simulink model "dual_hall_ideal_sincos"  (R2024b)
settings: Solver=ode4  StartTime=0.0  StopTime=hall_t_stop_s  FixedStep=hall_ts_sim_s  RelTol=1e-3
model workspace (MAT data in the model file):
  hall_adc_bits = 16
  hall_amp_c_v = 0.85
  hall_amp_s_v = 1
  hall_amp_v = 1
  hall_f_mag_hz = 3
  hall_f_mech_hz = 0.5
  hall_magnet_od_mm = 18
  hall_mech_speed_rpm = 30
  hall_offset_c_actual_v = 1.57
  hall_offset_err_c_v = -0.08
  hall_offset_err_s_v = 0.05
  hall_offset_s_actual_v = 1.7
  hall_offset_v = 1.65
  hall_omega_mech_rad_s = 3.14159265359
  hall_phase_err_deg = 5
  hall_phase_err_rad = 0.0872664625997
  hall_pole_pairs = 6
  hall_t_stop_s = 2
  hall_theta0_rad = 0
  hall_ts_sim_s = 0.0001
  hall_vref_v = 3.3
settings Model: Creator=26683  LastModifiedBy=26683

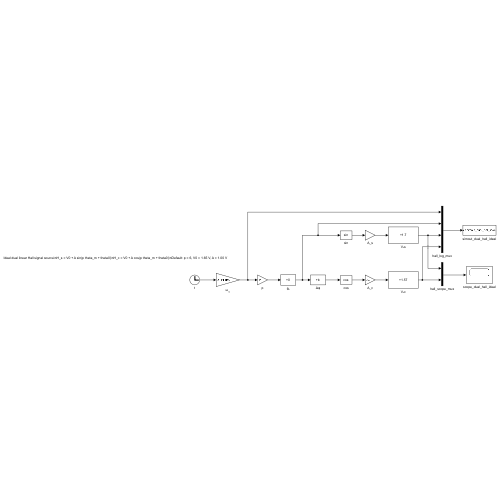
[thumbnail: Simulink's stored preview of the top-level diagram]
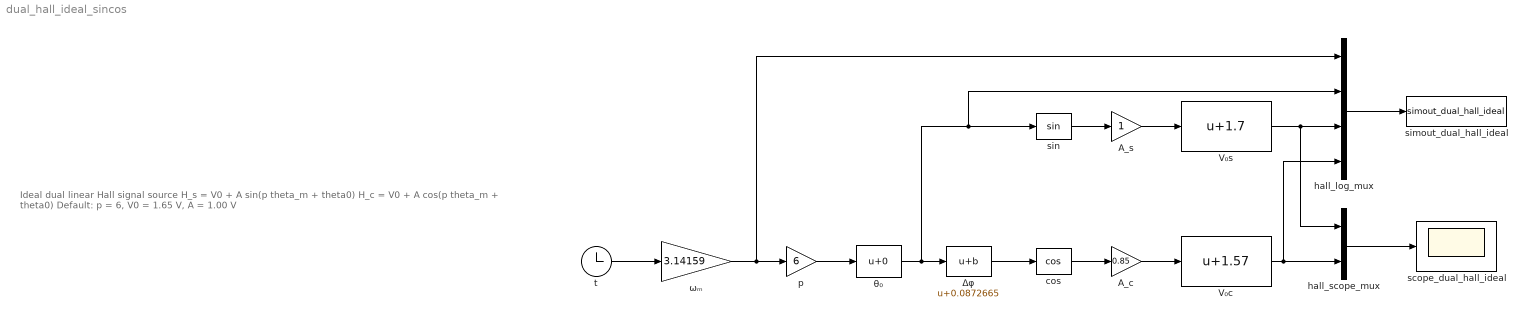
== system dual_hall_ideal_sincos ==
  note: Ideal dual linear Hall signal source\nH_s = V0 + A sin(p theta_m + theta0)\nH_c = V0 + A cos(p theta_m + theta0)\nDefault: p = 6, V0 = 1.65 V, A = 1.00 V
  A_c : Gain  Gain=0.85
  A_s : Gain
  V₀c : Bias  Bias=1.57  SaturateOnIntegerOverflow=off
  V₀s : Bias  Bias=1.7  SaturateOnIntegerOverflow=off
  cos : Trigonometry  Operator=cos
  hall_log_mux : Mux
  hall_scope_mux : Mux  Inputs=2
  p : Gain  Gain=6
  scope_dual_hall_ideal : Scope
  simout_dual_hall_ideal : ToWorkspace  VariableName=simout_dual_hall_ideal  SaveFormat=Structure With Time  SampleTime=-1
  sin : Trigonometry
  t : Clock
  Δφ : Bias  Bias=0.0872665  SaturateOnIntegerOverflow=off
  θ₀ : Bias  SaturateOnIntegerOverflow=off
  ωₘ : Gain  Gain=3.14159
  wires:
  t/1 -> ωₘ/1
  θ₀/1 -> Δφ/1, sin/1, hall_log_mux/2
  p/1 -> θ₀/1
  ωₘ/1 -> p/1, hall_log_mux/1
  A_c/1 -> V₀c/1
  A_s/1 -> V₀s/1
  cos/1 -> A_c/1
  V₀s/1 -> hall_scope_mux/1, hall_log_mux/3
  sin/1 -> A_s/1
  hall_log_mux/1 -> simout_dual_hall_ideal/1
  V₀c/1 -> hall_log_mux/4, hall_scope_mux/2
  hall_scope_mux/1 -> scope_dual_hall_ideal/1
  Δφ/1 -> cos/1
